simulink model "second_loop_v2"  (R2019b)
settings: Solver=VariableStepAuto  StartTime=0.0  StopTime=10  RelTol=1e-3
values from neighbouring files (symbols this model uses):
  K = [66.2259572254 -60.3086645892 5.93307364323 -20.4157003719]    [lqr_K.mat]    (also in lqr_controller.m = lqr(sys,Q,R); swmain.m = lqr_controller(sys2))
  sys2 = get_system2(params)    [swmain.m]
  Ts = 0.1    [swmain.m]
  wc = 2*f*pi    (= 12.5663706144)    [swmain.m]
  x_d = desired_state(theta_d, params)    [swmain.m]
settings Model: Creator=martijndebeuf  LastModifiedBy=martijndebeuf

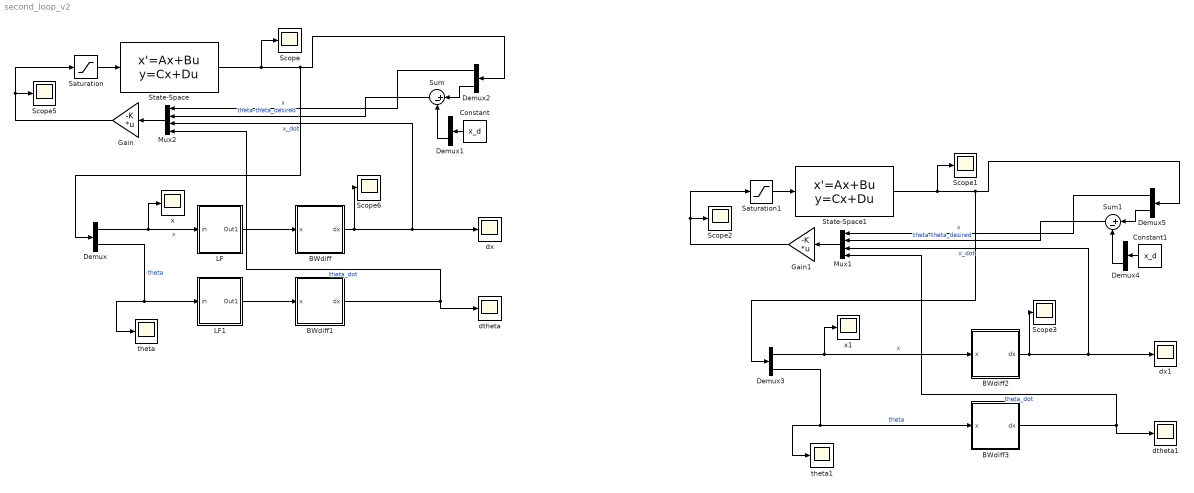
== system second_loop_v2 ==
  BWdiff : Subsystem
  BWdiff1 : Subsystem
  BWdiff2 : Subsystem
  BWdiff3 : Subsystem
  Constant : Constant  Value=x_d
  Constant1 : Constant  Value=x_d
  Demux{,1..5} (6 alike) : Demux  Outputs=2
  Gain : Gain  Gain=-K  Multiplication=Matrix(K*u) (u vector)
  Gain1 : Gain  Gain=-K  Multiplication=Matrix(K*u) (u vector)
  LF : Subsystem
  LF1 : Subsystem
  Mux1 : Mux
  Mux2 : Mux
  Saturation : Saturate  UpperLimit=5  LowerLimit=-5
  Saturation1 : Saturate  UpperLimit=5  LowerLimit=-5
  Scope{,1..3,5..6} (6 alike) : Scope
  State-Space : StateSpace  A=sys2.A  B=sys2.B  C=sys2.C  D=sys2.D  InitialCondition=initial_conditions'
  State-Space1 : StateSpace  A=sys2.A  B=sys2.B  C=sys2.C  D=sys2.D  InitialCondition=initial_conditions'
  Sum : Sum  Inputs=|+-
  Sum1 : Sum  Inputs=|+-
  dtheta : Scope
  dtheta1 : Scope
  dx : Scope
  dx1 : Scope
  theta : Scope
  theta1 : Scope
  x : Scope
  x1 : Scope
  wires:
  Demux/1 -> LF/1(in), x/1  "x"
  Demux/2 -> LF1/1(in), theta/1  "theta"
  BWdiff/1(dx) -> Mux2/3, dx/1, Scope6/1  "x_dot"
  BWdiff1/1(dx) -> Mux2/4, dtheta/1  "theta_dot"
  Saturation/1 -> State-Space/1
  Mux2/1 -> Gain/1
  Constant/1 -> Demux1/1
  Demux1/2 -> Sum/2
  Demux2/2 -> Sum/1
  Sum/1 -> Mux2/2  "theta-theta_desired"
  Demux2/1 -> Mux2/1  "x"
  State-Space/1 -> Scope/1, Demux/1, Demux2/1
  Gain/1 -> Scope5/1, Saturation/1
  LF/1(Out1) -> BWdiff/1(x)
  LF1/1(Out1) -> BWdiff1/1(x)
  Demux5/1 -> Mux1/1  "x"
  BWdiff3/1(dx) -> Mux1/4, dtheta1/1  "theta_dot"
  Sum1/1 -> Mux1/2  "theta-theta_desired"
  State-Space1/1 -> Scope1/1, Demux3/1, Demux5/1
  Mux1/1 -> Gain1/1
  Gain1/1 -> Scope2/1, Saturation1/1
  Demux3/1 -> BWdiff2/1(x), x1/1  "x"
  BWdiff2/1(dx) -> Mux1/3, dx1/1, Scope3/1  "x_dot"
  Demux3/2 -> BWdiff3/1(x), theta1/1  "theta"
  Demux4/2 -> Sum1/2
  Demux5/2 -> Sum1/1
  Saturation1/1 -> State-Space1/1
  Constant1/1 -> Demux4/1

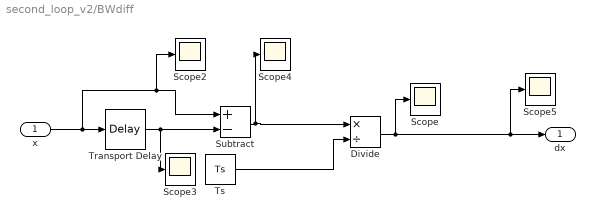
== system second_loop_v2/BWdiff ==
  x : Inport
  Divide : Product  Inputs=*/
  Scope{,2..5} (5 alike) : Scope
  Subtract : Sum  Inputs=+-
  Transport Delay : TransportDelay  DelayTime=Ts
  Ts : Constant  Value=Ts
  dx : Outport
  wires:
  Transport Delay/1 -> Scope3/1, Subtract/2
  Ts/1 -> Divide/2
  x/1 -> Transport Delay/1, Scope2/1, Subtract/1
  Subtract/1 -> Divide/1, Scope4/1
  Divide/1 -> Scope5/1, dx/1, Scope/1

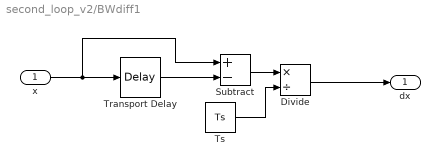
== system second_loop_v2/BWdiff1 ==
  x : Inport
  Divide : Product  Inputs=*/
  Subtract : Sum  Inputs=+-
  Transport Delay : TransportDelay  DelayTime=Ts
  Ts : Constant  Value=Ts
  dx : Outport
  wires:
  Ts/1 -> Divide/2
  Subtract/1 -> Divide/1
  x/1 -> Transport Delay/1, Subtract/1
  Divide/1 -> dx/1
  Transport Delay/1 -> Subtract/2

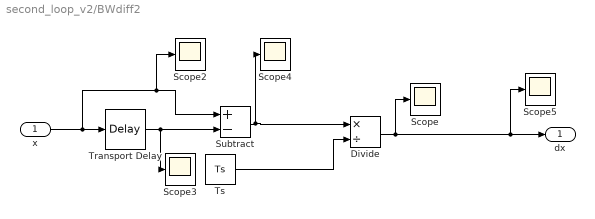
== system second_loop_v2/BWdiff2 ==
  x : Inport
  Divide : Product  Inputs=*/
  Scope{,2..5} (5 alike) : Scope
  Subtract : Sum  Inputs=+-
  Transport Delay : TransportDelay  DelayTime=Ts
  Ts : Constant  Value=Ts
  dx : Outport
  wires:
  Transport Delay/1 -> Scope3/1, Subtract/2
  Ts/1 -> Divide/2
  x/1 -> Transport Delay/1, Scope2/1, Subtract/1
  Subtract/1 -> Divide/1, Scope4/1
  Divide/1 -> Scope5/1, dx/1, Scope/1

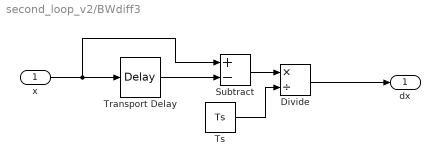
== system second_loop_v2/BWdiff3 ==
  x : Inport
  Divide : Product  Inputs=*/
  Subtract : Sum  Inputs=+-
  Transport Delay : TransportDelay  DelayTime=Ts
  Ts : Constant  Value=Ts
  dx : Outport
  wires:
  Ts/1 -> Divide/2
  Subtract/1 -> Divide/1
  x/1 -> Transport Delay/1, Subtract/1
  Divide/1 -> dx/1
  Transport Delay/1 -> Subtract/2

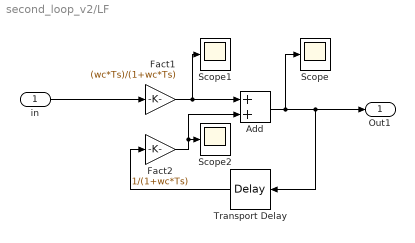
== system second_loop_v2/LF ==
  in : Inport
  Add : Sum
  Fact1 : Gain  Gain=(wc*Ts)/(1+wc*Ts)
  Fact2 : Gain  Gain=1/(1+wc*Ts)
  Scope : Scope
  Scope1 : Scope
  Scope2 : Scope
  Transport Delay : TransportDelay  DelayTime=Ts
  Out1 : Outport
  wires:
  Fact2/1 -> Scope2/1, Add/2
  Fact1/1 -> Scope1/1, Add/1
  in/1 -> Fact1/1
  Add/1 -> Scope/1, Transport Delay/1, Out1/1
  Transport Delay/1 -> Fact2/1

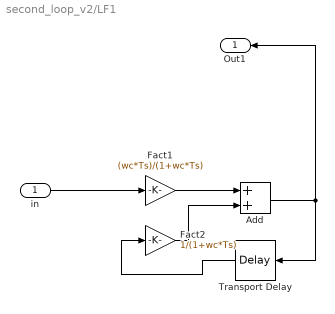
== system second_loop_v2/LF1 ==
  in : Inport
  Add : Sum
  Fact1 : Gain  Gain=(wc*Ts)/(1+wc*Ts)
  Fact2 : Gain  Gain=1/(1+wc*Ts)
  Transport Delay : TransportDelay  DelayTime=Ts
  Out1 : Outport
  wires:
  Add/1 -> Transport Delay/1, Out1/1
  Fact2/1 -> Add/2
  Fact1/1 -> Add/1
  in/1 -> Fact1/1
  Transport Delay/1 -> Fact2/1
